simulink model "ofdmexample1"  (R2017a)
settings: Solver=FixedStepDiscrete  StartTime=0.0  StopTime=0.1  RelTol=1e-3
PostLoadFcn:
  | prm80216d.blkh = []; prm80216d.action = 'init';
  | commwman80216d_init(prm80216d.blkh, prm80216d.action);
  | if isempty(ans), clear ans; end
StartFcn:
  | if isempty(ans), clear ans; end
undefined symbols (not defined in the file): idx, magnitude
libraries: commwman80216d_lib x49, dspsigops x24, commcnvcod2 x14, dspindex x4, commdigbbndpm3 x3, dspsolvers x2, simulink x2, commrflib2 x2, commofdm x2, commsink2 x1, commblksprivate x1, dspmtrx3 x1
(part 1 of 2)
Description:
  | IEEE 802.16-2004 WirelessMAN-OFDM PHY Downlink model
settings Model: FPTRunName=Active  ExtModeAutoUpdateStatusClock=off  Creator=The MathWorks, Inc.  LastModifiedBy=max
settings DataIOCC: LimitDataPoints=on  SaveFormat=Array
settings OptimizationCC: ExpressionDepthLimit=2147483647  InitFltsAndDblsToZero=on  EfficientMapNaN2IntZero=off  LifeSpan=inf
settings DebuggingCC: UnderspecifiedInitializationDetection=Classic  MergeDetectMultiDrivingBlocksExec=none  FcnCallInpInsideContextMsg=warning  AllowSymbolicDim=off  StateNameClashWarn=warning  SFUnexpectedBacktrackingDiag=warning  SFNoUnconditionalDefaultTransitionDiag=warning  SFExecutionAtInitializationDiag=none
settings HardwareCC: ProdBitPerPointer=32  ProdBitPerSizeT=32  ProdBitPerPtrDiffT=32  ProdLargestAtomicFloat=None  ProdIntDivRoundTo=Undefined  ProdEndianess=Unspecified  ProdWordSize=32  ProdHWDeviceType=32-bit Generic
settings ModelReferenceCC: PropagateSignalLabelsOutOfModel=off
settings RTWCC: RetainRTWFile=on
settings GRTTargetCC: TargetFcnLib=ansi_tfl_tmw_new.mat  TargetLangStandard=C89/C90 (ANSI)  GeneratePreprocessorConditionals=Disable all  CombineOutputUpdateFcns=off  GRTInterface=on
settings ConfigComp: CovMetricSettings=dw  CovHtmlReporting=on  CovSaveCumulativeToWorkspaceVar=on  CovSaveSingleToWorkspaceVar=on  CovExternalEMLEnable=off  CovSFcnEnable=off

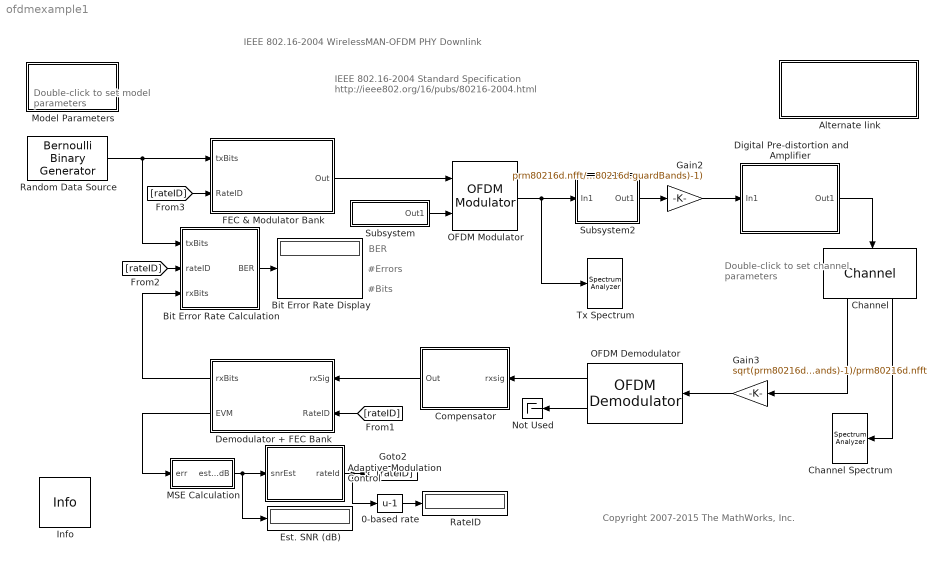
== system ofdmexample1 ==
  note: IEEE 802.16-2004 WirelessMAN-OFDM PHY Downlink
  note: BER
  note: #Bits
  note: #Errors
  note: Double-click to set
      | channel parameters
  note: Double-click to
      | set model parameters
  note: IEEE 802.16-2004 Standard Specification
      | http://ieee802.org/16/pubs/80216-2004.html
  note: Copyright 2007-2015 The MathWorks, Inc.
  0-based rate : Bias  Bias=-1
  Adaptive Modulation Control : Subsystem  mask{thres=prm80216d.thresholds}
      mask prompts: thres "Low-SNR thresholds (dB):"
      mask init:
      | snrUp = [thres inf];
      | snrDown = [-inf thres];
      mask Display: disp('Adaptive\nRate\nControl')
  Alternate link : Subsystem
      settings: OpenFcn=commwman80216dstbc;
      mask Display: disp('Double-click to open\n link model with\nSpace-Time Block Coding');
  Bit Error Rate Calculation : Subsystem
      mask Display: disp('Bit Error Rate\nCalculation');
  Bit Error Rate Display : Display
  Channel : commwman80216d_lib/Channel  fadingMode=Frequency-selective fading  K=4  maxDoppler=0.5  pathDelays=[0 0.4 0.9]*1e-6  pathGains=[0 -15 -20]  SNRdB=30
      settings: SourceProductName=Communications System Toolbox  SourceProductBaseCode=CM
  Channel Spectrum : SpectrumAnalyzer
  Compensator : Subsystem
      mask Display: disp('Gain & Phase\nCompensator');
  Demodulator + FEC Bank : Subsystem
      mask Display: disp('Demodulator\n& FEC Bank');
  Digital Pre-distortion and Amplifier : Subsystem
      mask Display: disp('Digital\nPre-Distortion and\nNonlinear\nAmplifier')
  Est. SNR (dB) : Display
  FEC & Modulator Bank : Subsystem
      mask Display: disp('FEC & \nModulator Bank');
  Gain2 : Gain  Gain=prm80216d.nfft/sqrt(prm80216d.nfft-sum(prm80216d.guardBands)-1)
  Gain3 : Gain  Gain=sqrt(prm80216d.nfft-sum(prm80216d.guardBands)-1)/prm80216d.nfft
  Info : commblksprivate/Info  SystemSampleTime=-1
      settings: SourceProductName=Communications System Toolbox  SourceProductBaseCode=CM
  MSE Calculation : Subsystem
      mask Display: disp('SNR\nEstimation')
  Model Parameters : Subsystem  mask(Model Parameters){chanBW=3.5, numSym=1, g=1/8, nonlinCtrl=Disabled, dpdCtrl=Disabled, thresh=[4 10 12 19 22 28]}
      mask prompts: chanBW "Channel bandwidth (MHz):"; numSym "Number of OFDM symbols per burst:"; g "Cyclic prefix factor (G):"; nonlinCtrl "Amplifier nonlinearity:"; dpdCtrl "Digital pre-distortion:"; thresh "Low SNR thresholds for rate control (dB):"
      mask help: Specifies model parameters for a simulation run.
      mask init:
      | numPreSym = 1; % number of preamble OFDM symbols
      | 
      | % If the nonlinearity is turned off, then turn off the digital
      | % pre-distortion
      | if nonlinCtrl == 1  % disabled
      |     dpdCtrl = 1;
      | end
      | 
      | myException = commwman80216d_init(gcbh, 'init', chanBW, ...
      |     numSym, numPreSym, g, thresh);
      | 
      | if ~isempty(myException)
      |     errordlg(myException.msg);
      | end
      mask Help: helpview(commdhelp);
      mask TypeOptions g: 1/4 | 1/8 | 1/16 | 1/32
      mask TypeOptions nonlinCtrl: Disabled | Moderate (correctable by pre-distortion) | Severe (uncorrectable by pre-distortion)
      mask Callback nonlinCtrl: commwman80216d_init(gcbh, 'cbShowHidePreDistortion');
      mask TypeOptions dpdCtrl: Disabled | Enabled
      mask Display: disp('Model\nParameters');
  Not Used : Terminator
  OFDM Demodulator : commofdm/OFDM Demodulator  FFTLength=prm80216d.nfft  NumGuardBandCarriers=prm80216d.guardBands  RemoveDCCarrier=on  PilotOutputPort=on  PilotCarrierIndices=prm80216d.pilotIndices + prm80216d.nfft/2 + 1  CyclicPrefixLength=prm80216d.CPLen  NumSymbols=prm80216d.totOFDMSym  NumReceiveAntennas=1  SimulateUsing=Interpreted execution
      settings: SourceProductName=Communications System Toolbox  SourceProductBaseCode=CM
  OFDM Modulator : commofdm/OFDM Modulator  FFTLength=prm80216d.nfft  NumGuardBandCarriers=prm80216d.guardBands  InsertDCNull=on  PilotInputPort=on  PilotCarrierIndices=prm80216d.pilotIndices + prm80216d.nfft/2 + 1  CyclicPrefixLength=prm80216d.CPLen  Windowing=off  WindowLength=1  NumSymbols=prm80216d.numOFDMSymbols  NumTransmitAntennas=1  SimulateUsing=Interpreted execution
      settings: SourceProductName=Communications System Toolbox  SourceProductBaseCode=CM
  Random Data Source : commrandsrc3/Bernoulli Binary Generator  ProbabilityOfZero=0.5  SeedSource=Parameter  Seed=61  SampleTime=prm80216d.minBitPeriod  SamplesPerFrame=prm80216d.maxUncBitsPerBlk*prm80216d.numOFDMSymbols  OutputDataType=boolean  SimulateUsing=Interpreted execution
  RateID : Display
  Subsystem : Subsystem
      mask Display: disp('Pilot')
  Subsystem2 : Subsystem
      mask Display: disp('Preamble\nPacking');
  Tx Spectrum : SpectrumAnalyzer
  wires:
  Gain2/1 -> Digital Pre-distortion and Amplifier/1(In1)
  Random Data Source/1 -> Bit Error Rate Calculation/1(txBits), FEC & Modulator Bank/1(txBits)
  Bit Error Rate Calculation/1(BER) -> Bit Error Rate Display/1
  Demodulator + FEC Bank/2(EVM) -> MSE Calculation/1(err)
  [rateID] -> FEC & Modulator Bank/2(RateID)
  [rateID] -> Demodulator + FEC Bank/2(RateID)
  [rateID] -> Bit Error Rate Calculation/2(rateID)
  Demodulator + FEC Bank/1(rxBits) -> Bit Error Rate Calculation/3(rxBits)
  Adaptive Modulation Control/1(rateId) -> [rateID], 0-based rate/1
  MSE Calculation/1(estSNRdB) -> Adaptive Modulation Control/1(snrEst), Est. SNR (dB)/1
  0-based rate/1 -> RateID/1
  Digital Pre-distortion and Amplifier/1(Out1) -> Channel/1
  Channel/1 -> Gain3/1
  Channel/2 -> Channel Spectrum/1
  Gain3/1 -> OFDM Demodulator/1
  OFDM Demodulator/1 -> Compensator/1(rxsig)
  OFDM Demodulator/2 -> Not Used/1
  Subsystem/1(Out1) -> OFDM Modulator/2
  OFDM Modulator/1 -> Subsystem2/1(In1), Tx Spectrum/1
  FEC & Modulator Bank/1(Out) -> OFDM Modulator/1
  Compensator/1(Out) -> Demodulator + FEC Bank/1(rxSig)
  Subsystem2/1(Out1) -> Gain2/1

== system ofdmexample1/Adaptive Modulation Control ==
  note: dec by 1
  note: inc by 1
  snrEst : Inport
  Add1 : Sum  Inputs=+-+  OutDataTypeStr=double
  Integer Delay : Delay  DelayLength=1  InitialCondition=1 % rateID 0 => BPSK
  Relational Operator : RelationalOperator  Operator=>  RndMeth=Nearest
  Relational Operator1 : RelationalOperator  Operator=<=  RndMeth=Nearest
  SNR down threshold : commwman80216d_lib/Select Value  vector=snrDown
      settings: SourceProductName=Communications System Toolbox  SourceProductBaseCode=CM
  SNR up threshold : commwman80216d_lib/Select Value  vector=snrUp
      settings: SourceProductName=Communications System Toolbox  SourceProductBaseCode=CM
  rateId : Outport
  wires:
  Add1/1 -> Integer Delay/1
  SNR down threshold/1 -> Relational Operator1/2
  SNR up threshold/1 -> Relational Operator/2
  Integer Delay/1 -> rateId/1, SNR up threshold/1, SNR down threshold/1, Add1/3
  Relational Operator1/1 -> Add1/2
  Relational Operator/1 -> Add1/1
  snrEst/1 -> Relational Operator1/1, Relational Operator/1

== system ofdmexample1/Alternate link ==

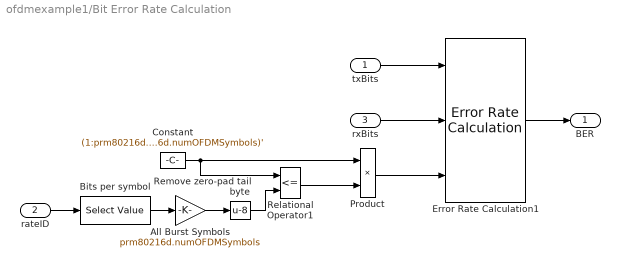
== system ofdmexample1/Bit Error Rate Calculation ==
  txBits : Inport
  rateID : Inport  Port=2
  rxBits : Inport  Port=3
  All Burst Symbols : Gain  Gain=prm80216d.numOFDMSymbols
  Bits per symbol : commwman80216d_lib/Select Value  vector=prm80216d.uncBlkSize*8
      settings: SourceProductName=Communications System Toolbox  SourceProductBaseCode=CM
  Constant : Constant  Value=(1:prm80216d.maxUncBitsPerBlk*prm80216d.numOFDMSymbols)'  VectorParams1D=off
  Error Rate Calculation1 : commsink2/Error Rate Calculation  N=0  st_delay=0  cp_mode=Select samples from port  subframe=1:(idx*8*prm80216d.numOFDMSymbols - 8)  PMode=Port  WsName=ErrorVec  RsMode2=off  stop=off  numErr=inf  maxBits=5e5
  Product : Product  SaturateOnIntegerOverflow=on  OutDataTypeStr=Inherit: Same as first input
  Relational Operator1 : RelationalOperator  Operator=<=  OutDataTypeStr=float('double')  RndMeth=Nearest  InputSameDT=on
  Remove zero-pad tail byte : Bias  Bias=-8
  BER : Outport
  wires:
  txBits/1 -> Error Rate Calculation1/1
  Error Rate Calculation1/1 -> BER/1
  rxBits/1 -> Error Rate Calculation1/2
  rateID/1 -> Bits per symbol/1
  Relational Operator1/1 -> Product/2
  Constant/1 -> Product/1, Relational Operator1/1
  All Burst Symbols/1 -> Remove zero-pad tail byte/1
  Product/1 -> Error Rate Calculation1/3
  Bits per symbol/1 -> All Burst Symbols/1
  Remove zero-pad tail byte/1 -> Relational Operator1/2

== system ofdmexample1/Compensator ==
  rxsig : Inport
  Compensator : Subsystem
      mask init:
      | a = [1:100; 1:100];
      mask Display: disp('Gain & Phase\nCompensator')
  Extract Nonzero Preamble Subcarriers : dspindex/Multiport Selector  rowsOrCols=Rows  idxCellArray=prm80216d.nonzeroPreambleIdxTx1  idxErrMode=Clip Index
  Training Preamble : Constant  Value=prm80216d.preambleTx1  VectorParams1D=off
  Out : Outport
  wires:
  Training Preamble/1 -> Extract Nonzero Preamble Subcarriers/1
  rxsig/1 -> Compensator/1(rxsig)
  Compensator/1(out) -> Out/1
  Extract Nonzero Preamble Subcarriers/1 -> Compensator/2(trainsig)

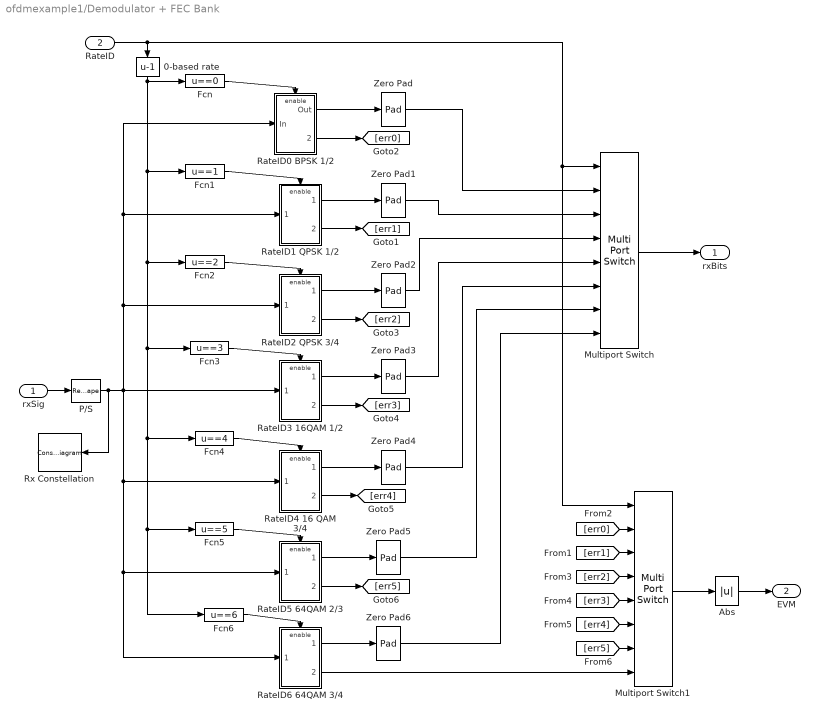
== system ofdmexample1/Demodulator + FEC Bank ==
  rxSig : Inport
  RateID : Inport  Port=2
  0-based rate : Bias  Bias=-1
  Abs : Abs  SaturateOnIntegerOverflow=on
  Fcn : Fcn  Expr=u==0
  Fcn1 : Fcn  Expr=u==1
  Fcn2 : Fcn  Expr=u==2
  Fcn3 : Fcn  Expr=u==3
  Fcn4 : Fcn  Expr=u==4
  Fcn5 : Fcn  Expr=u==5
  Fcn6 : Fcn  Expr=u==6
  Multiport Switch : MultiPortSwitch  Inputs=7  SaturateOnIntegerOverflow=on
  Multiport Switch1 : MultiPortSwitch  Inputs=7  SaturateOnIntegerOverflow=on
  P/S : Reshape  OutputDimensionality=Column vector (2-D)  OutputDimensions=[prm80216d.numDataSym, prm80216d.numOFDMSymbols]
  RateID0 BPSK 1/2 : Subsystem
  RateID1 QPSK 1/2 : Subsystem
  RateID2 QPSK 3/4 : Subsystem
  RateID3 16QAM 1/2 : Subsystem
  RateID4 16 QAM 3/4 : Subsystem
  RateID5 64QAM 2/3 : Subsystem
  RateID6 64QAM 3/4 : Subsystem
  Rx Constellation : ConstellationDiagram  Tag=ScatterPlot
  Zero Pad{,1..6} (7 alike) : dspsigops/Pad  padAlong=Columns  dimsToPad=1  valSrc=Specify via dialog  padVal=0  spec=Output size  padNumOutRowsSpecMethod=User-specified  numOutRows=prm80216d.maxUncBitsPerBlk*prm80216d.numOFDMSymbols  padNumOutColsSpecMethod=User-specified  numOutCols=1  isVarDimsMode=off  padBeginning=0  padEnd=0  outSizeMode=User-specified  outSize=1  padSigAt=End  trunc_flag=None  roundingMode=Floor  overflowMode=off  truncOrWrapMode=Truncate  wrap_flag=None
      settings: AttributesFormatString=\n  SourceProductName=DSP System Toolbox  SourceProductBaseCode=DS
  rxBits : Outport
  EVM : Outport  Port=2
  wires:
  RateID/1 -> Multiport Switch/1, Multiport Switch1/1, 0-based rate/1
  Multiport Switch/1 -> rxBits/1
  RateID0 BPSK 1/2/1(Out) -> Zero Pad/1
  RateID1 QPSK 1/2/1(Out1) -> Zero Pad1/1
  RateID2 QPSK 3/4/1(Out2) -> Zero Pad2/1
  RateID3 16QAM 1/2/1(Out3) -> Zero Pad3/1
  RateID4 16 QAM 3/4/1(Out4) -> Zero Pad4/1
  RateID5 64QAM 2/3/1(Out5) -> Zero Pad5/1
  RateID6 64QAM 3/4/1(Out6) -> Zero Pad6/1
  Fcn/1 -> RateID0 BPSK 1/2/Enable
  Fcn1/1 -> RateID1 QPSK 1/2/Enable
  Fcn2/1 -> RateID2 QPSK 3/4/Enable
  Fcn3/1 -> RateID3 16QAM 1/2/Enable
  Fcn4/1 -> RateID4 16 QAM 3/4/Enable
  Fcn5/1 -> RateID5 64QAM 2/3/Enable
  Fcn6/1 -> RateID6 64QAM 3/4/Enable
  Zero Pad/1 -> Multiport Switch/2
  Zero Pad2/1 -> Multiport Switch/4
  Zero Pad3/1 -> Multiport Switch/5
  Zero Pad4/1 -> Multiport Switch/6
  Zero Pad5/1 -> Multiport Switch/7
  Zero Pad6/1 -> Multiport Switch/8
  Multiport Switch1/1 -> Abs/1
  RateID6 64QAM 3/4/2(symerr) -> Multiport Switch1/8
  Abs/1 -> EVM/1
  0-based rate/1 -> Fcn/1, Fcn1/1, Fcn2/1, Fcn3/1, Fcn4/1, Fcn5/1, Fcn6/1
  RateID0 BPSK 1/2/2(symerr) -> [err0]
  RateID1 QPSK 1/2/2(symerr) -> [err1]
  RateID2 QPSK 3/4/2(symerr) -> [err2]
  RateID3 16QAM 1/2/2(symerr) -> [err3]
  RateID4 16 QAM 3/4/2(symerr) -> [err4]
  RateID5 64QAM 2/3/2(symerr) -> [err5]
  [err0] -> Multiport Switch1/2
  [err1] -> Multiport Switch1/3
  [err2] -> Multiport Switch1/4
  [err3] -> Multiport Switch1/5
  [err4] -> Multiport Switch1/6
  [err5] -> Multiport Switch1/7
  Zero Pad1/1 -> Multiport Switch/3
  rxSig/1 -> P/S/1
  P/S/1 -> Rx Constellation/1, RateID4 16 QAM 3/4/1(In4), RateID5 64QAM 2/3/1(In5), RateID6 64QAM 3/4/1(In6), RateID0 BPSK 1/2/1(In), RateID1 QPSK 1/2/1(In1), RateID2 QPSK 3/4/1(In2), RateID3 16QAM 1/2/1(In3)

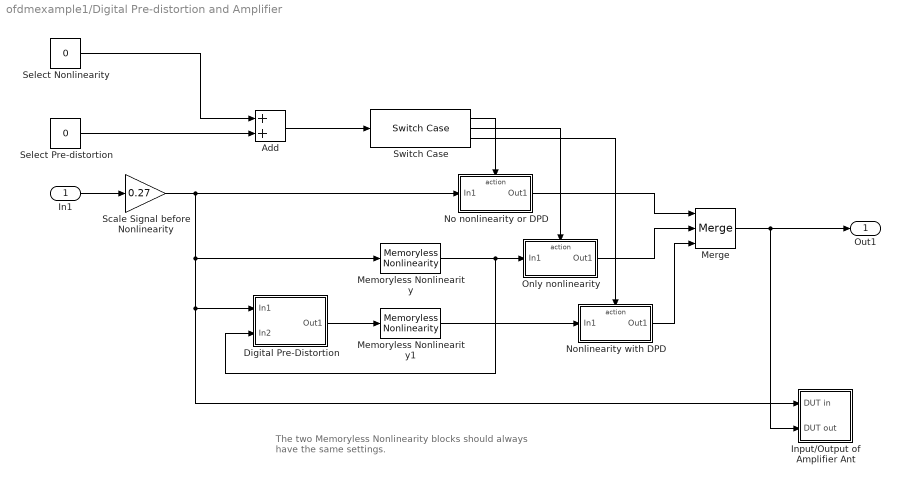
== system ofdmexample1/Digital Pre-distortion and Amplifier ==
  note: The two Memoryless Nonlinearity blocks should always
      | have the same settings.
  In1 : Inport
  Add : Sum
  Digital Pre-Distortion : Subsystem
      mask Display: disp('Digital\nPre-Distortion')
  Input/Output of Amplifier Ant : Subsystem
  Memoryless Nonlinearity : commrflib2/Memoryless Nonlinearity  model_select=Saleh model  linGaindB=0  GindB=0  iip3=30  am2pm=10  LPwrLimAMPM=10  UPwrLimAMPM=inf  amam=[2.1587 1.1517]  ampm=[4.0033 9.1040]  x=[8.1081 1.5413 6.5202 -0.0718]  y=[4.6645 2.0965 10.88 -0.003]  p=0.5  GoutdB=0  vsat=1
      settings: SourceProductName=Communications System Toolbox  SourceProductBaseCode=CM
  Memoryless Nonlinearity1 : commrflib2/Memoryless Nonlinearity  model_select=Saleh model  linGaindB=0  GindB=0  iip3=30  am2pm=10  LPwrLimAMPM=10  UPwrLimAMPM=inf  amam=[2.1587 1.1517]  ampm=[4.0033 9.1040]  x=[8.1081 1.5413 6.5202 -0.0718]  y=[4.6645 2.0965 10.88 -0.003]  p=0.5  GoutdB=0  vsat=1
      settings: SourceProductName=Communications System Toolbox  SourceProductBaseCode=CM
  Merge : Merge  Inputs=3
  No nonlinearity or DPD : Subsystem  TreatAsAtomicUnit=on
  Nonlinearity with DPD : Subsystem  TreatAsAtomicUnit=on
  Only nonlinearity : Subsystem  TreatAsAtomicUnit=on
  Scale Signal before Nonlinearity : Gain  Gain=0.27
  Select Nonlinearity : Constant  Value=0
  Select Pre-distortion : Constant  Value=0
  Switch Case : SwitchCase  CaseConditions={0,1,2}  ShowDefaultCase=off
  Out1 : Outport
  wires:
  Scale Signal before Nonlinearity/1 -> No nonlinearity or DPD/1(In1), Input/Output of Amplifier Ant/1(DUT in), Digital Pre-Distortion/1(In1), Memoryless Nonlinearity/1
  Digital Pre-Distortion/1(Out1) -> Memoryless Nonlinearity1/1
  Select Pre-distortion/1 -> Add/2
  Add/1 -> Switch Case/1
  Select Nonlinearity/1 -> Add/1
  In1/1 -> Scale Signal before Nonlinearity/1
  Memoryless Nonlinearity1/1 -> Nonlinearity with DPD/1(In1)
  Memoryless Nonlinearity/1 -> Only nonlinearity/1(In1), Digital Pre-Distortion/2(In2)
  Merge/1 -> Input/Output of Amplifier Ant/2(DUT out), Out1/1
  Switch Case/1 -> No nonlinearity or DPD/Action
  Switch Case/2 -> Only nonlinearity/Action
  Switch Case/3 -> Nonlinearity with DPD/Action
  No nonlinearity or DPD/1(Out1) -> Merge/1
  Only nonlinearity/1(Out1) -> Merge/2
  Nonlinearity with DPD/1(Out1) -> Merge/3

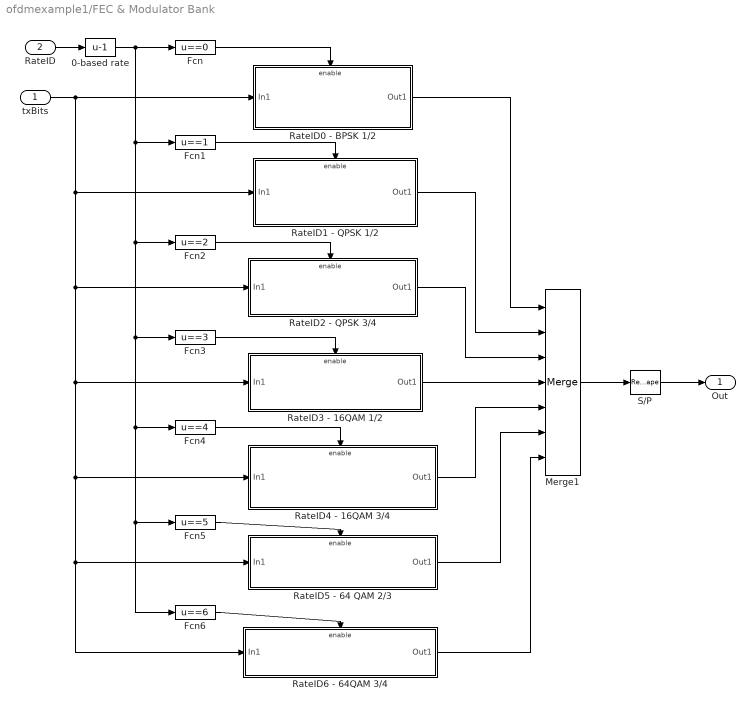
== system ofdmexample1/FEC & Modulator Bank ==
  txBits : Inport
  RateID : Inport  Port=2
  0-based rate : Bias  Bias=-1
  Fcn : Fcn  Expr=u==0
  Fcn1 : Fcn  Expr=u==1
  Fcn2 : Fcn  Expr=u==2
  Fcn3 : Fcn  Expr=u==3
  Fcn4 : Fcn  Expr=u==4
  Fcn5 : Fcn  Expr=u==5
  Fcn6 : Fcn  Expr=u==6
  Merge1 : Merge  Inputs=7
  RateID0 - BPSK 1/2 : Subsystem
  RateID1 - QPSK 1/2 : Subsystem
  RateID2 - QPSK 3/4 : Subsystem
  RateID3 - 16QAM 1/2 : Subsystem
  RateID4 - 16QAM 3/4 : Subsystem
  RateID5 - 64 QAM 2/3 : Subsystem
  RateID6 - 64QAM 3/4 : Subsystem
  S/P : Reshape  OutputDimensionality=Customize  OutputDimensions=[prm80216d.numDataCarriers, prm80216d.numOFDMSymbols]
  Out : Outport
  wires:
  RateID0 - BPSK 1/2/1(Out1) -> Merge1/1
  RateID1 - QPSK 1/2/1(Out1) -> Merge1/2
  RateID2 - QPSK 3/4/1(Out1) -> Merge1/3
  RateID3 - 16QAM 1/2/1(Out1) -> Merge1/4
  RateID4 - 16QAM 3/4/1(Out1) -> Merge1/5
  RateID5 - 64 QAM 2/3/1(Out1) -> Merge1/6
  RateID6 - 64QAM 3/4/1(Out1) -> Merge1/7
  txBits/1 -> RateID5 - 64 QAM 2/3/1(In1), RateID6 - 64QAM 3/4/1(In1), RateID4 - 16QAM 3/4/1(In1), RateID3 - 16QAM 1/2/1(In1), RateID2 - QPSK 3/4/1(In1), RateID1 - QPSK 1/2/1(In1), RateID0 - BPSK 1/2/1(In1)
  RateID/1 -> 0-based rate/1
  Fcn/1 -> RateID0 - BPSK 1/2/Enable
  Fcn1/1 -> RateID1 - QPSK 1/2/Enable
  Fcn2/1 -> RateID2 - QPSK 3/4/Enable
  Fcn3/1 -> RateID3 - 16QAM 1/2/Enable
  Fcn4/1 -> RateID4 - 16QAM 3/4/Enable
  Fcn5/1 -> RateID5 - 64 QAM 2/3/Enable
  Fcn6/1 -> RateID6 - 64QAM 3/4/Enable
  0-based rate/1 -> Fcn4/1, Fcn5/1, Fcn6/1, Fcn3/1, Fcn2/1, Fcn1/1, Fcn/1
  Merge1/1 -> S/P/1
  S/P/1 -> Out/1

== system ofdmexample1/MSE Calculation ==
  err : Inport
  Math Function2 : Math  Operator=reciprocal  SaturateOnIntegerOverflow=on
  Matrix Square : dspmtrx3/Matrix Square  OutMin=[]  OutMax=[]
      settings: SourceProductName=DSP System Toolbox  SourceProductBaseCode=DS
  RMS : dspstat3/RMS  run=off  directionMode=Each column  dimension=1  InputProcessing=Columns as channels (frame based)  reset_popup=None
  dB Conversion : dspmathops/dB Conversion  dBtype=dB  intype=Power  R=1  fuzz=on
      settings: SourceProductName=DSP System Toolbox
  estSNRdB : Outport
  wires:
  dB Conversion/1 -> estSNRdB/1
  err/1 -> RMS/1
  RMS/1 -> Matrix Square/1
  Math Function2/1 -> dB Conversion/1
  Matrix Square/1 -> Math Function2/1

== system ofdmexample1/Model Parameters ==
  note: This subsystem is empty.
      | It is used for setting parameter values (in the mask).

== system ofdmexample1/Subsystem ==
  Gain{,1,3..4} (4 alike) : Gain  Gain=-1
  Input Packing : Concatenate  NumInputs=8  Mode=Multidimensional array
  Pilots : commwman80216d_lib/Pilot Generator  link=Downlink  ts=prm80216d.maxUncBitsPerBlk*prm80216d.minBitPeriod  numSym=prm80216d.numOFDMSymbols  shift=prm80216d.numPreamOFDMSymbols
      settings: SourceProductName=Communications System Toolbox  SourceProductBaseCode=CM
  Out1 : Outport
  wires:
  Gain/1 -> Input Packing/4
  Pilots/1 -> Input Packing/1, Gain1/1, Input Packing/3, Gain/1, Gain3/1, Gain4/1, Input Packing/7, Input Packing/8
  Gain3/1 -> Input Packing/5
  Gain1/1 -> Input Packing/2
  Gain4/1 -> Input Packing/6
  Input Packing/1 -> Out1/1

== system ofdmexample1/Subsystem2 ==
  In1 : Inport
  Insert Preamble : Concatenate  Mode=Multidimensional array
  Subsystem1 : Subsystem
      mask Display: disp('Preamble')
  Out1 : Outport
  wires:
  In1/1 -> Insert Preamble/2
  Insert Preamble/1 -> Out1/1
  Subsystem1/1(Out) -> Insert Preamble/1

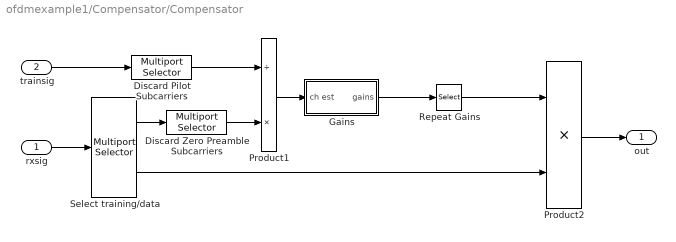
== system ofdmexample1/Compensator/Compensator ==
  rxsig : Inport
  trainsig : Inport  Port=2
  Discard Pilot Subcarriers : dspindex/Multiport Selector  rowsOrCols=Rows  idxCellArray=prm80216d.preambleEqIdxTx1  idxErrMode=Clip Index
  Discard Zero Preamble Subcarriers : dspindex/Multiport Selector  rowsOrCols=Rows  idxCellArray=prm80216d.dataEqIdxTx1  idxErrMode=Clip Index
  Gains : Subsystem
  Product1 : Product  Inputs=/*  SaturateOnIntegerOverflow=on  OutDataTypeStr=Inherit: Same as first input
  Product2 : Product  Inputs=**  SaturateOnIntegerOverflow=on  OutDataTypeStr=Inherit: Same as first input
  Repeat Gains : Selector  NumberOfDimensions=2  InputPortWidth=53  IndexOptions=Index vector (dialog),Select all  Indices=kron(1:prm80216d.numDataCarriers/2, [1 1]),-1  OutputSizes=1
  Select training/data : dspindex/Multiport Selector  rowsOrCols=Columns  idxCellArray={1:prm80216d.numPreamOFDMSymbols, prm80216d.numPreamOFDMSymbols+1:prm80216d.totOFDMSym}  idxErrMode=Clip Index
  out : Outport
  wires:
  Select training/data/1 -> Discard Zero Preamble Subcarriers/1
  Product2/1 -> out/1
  Product1/1 -> Gains/1(ch est)
  Gains/1(gains) -> Repeat Gains/1
  rxsig/1 -> Select training/data/1
  Repeat Gains/1 -> Product2/1
  Select training/data/2 -> Product2/2
  trainsig/1 -> Discard Pilot Subcarriers/1
  Discard Zero Preamble Subcarriers/1 -> Product1/2
  Discard Pilot Subcarriers/1 -> Product1/1

== system ofdmexample1/Demodulator + FEC Bank/RateID0 BPSK 1//2 ==
  In : Inport
  Enable : EnablePort  StatesWhenEnabling=reset  PropagateVarSize=During execution
  BPSK Demodulator : commdigbbndpm3/BPSK Demodulator Baseband  DecType=Hard decision  VarSource=Dialog  Variance=1  Ph=0  outDtype=boolean  derotateFactorWordLen=16  derotateFactorDataTypeStr=Inherit: Same word length as input  derotateFactorLastDataTypeStr=Inherit: Same word length as input
  BPSK Modulator : commdigbbndpm3/BPSK Modulator Baseband  Ph=0  outDtype=double  outWordLen=16  outUDDataType=sfix(16)  outFracLenMode=Best precision  outFracLen=15  outDataTypeStr=double  outLastDataTypeStr=double
  Deinterleaver : commwman80216d_lib/Deinterleaver  numSubCh=16  Ncbps1=192  Ncbps2=96  Ncbps3=48  Ncbps4=24  Ncbps5=12  Ncpc=1  numSym=prm80216d.numOFDMSymbols
      settings: SourceProductName=Communications System Toolbox  SourceProductBaseCode=CM
  Sum : Sum  Inputs=|+-  SaturateOnIntegerOverflow=on
  Viterbi Decoder : commcnvcod2/Viterbi Decoder  trellis=poly2trellis(7, [171 133])  isPunctured=off  punctureVector=reshape([1 0 1 0 1;1 1 0 1 0],10,1)  erasures=off  dectype=Hard decision  nsdecb=4  runSigValErrCheck=off  tbdepth=34  opmode=Truncated  reset=off  delayedResetAction=off  smWordLength=16  outDataType=boolean
      settings: SourceProductName=Communications System Toolbox  SourceProductBaseCode=CM
  Out : Outport
  symerr : Outport  Port=2  OutputWhenDisabled=reset  InitialOutput=0
  wires:
  Sum/1 -> symerr/1
  In/1 -> BPSK Demodulator/1, Sum/2
  BPSK Demodulator/1 -> Deinterleaver/1, BPSK Modulator/1
  Deinterleaver/1 -> Viterbi Decoder/1
  Viterbi Decoder/1 -> Out/1
  BPSK Modulator/1 -> Sum/1

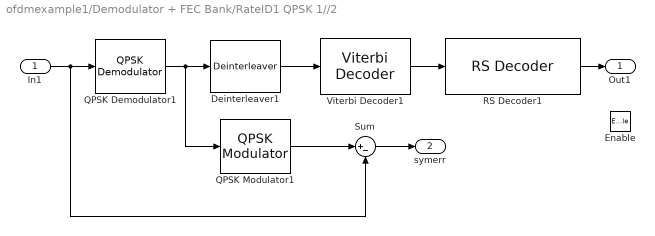
== system ofdmexample1/Demodulator + FEC Bank/RateID1 QPSK 1//2 ==
  In1 : Inport
  Enable : EnablePort  StatesWhenEnabling=reset  PropagateVarSize=During execution
  Deinterleaver1 : commwman80216d_lib/Deinterleaver  numSubCh=16  Ncbps1=384  Ncbps2=96  Ncbps3=48  Ncbps4=24  Ncbps5=12  Ncpc=2  numSym=prm80216d.numOFDMSymbols
      settings: SourceProductName=Communications System Toolbox  SourceProductBaseCode=CM
  QPSK Demodulator1 : commwman80216d_lib/QPSK Demodulator  SystemSampleTime=-1
      settings: SourceProductName=Communications System Toolbox  SourceProductBaseCode=CM
  QPSK Modulator1 : commwman80216d_lib/QPSK Modulator  SystemSampleTime=-1
      settings: SourceProductName=Communications System Toolbox  SourceProductBaseCode=CM
  RS Decoder1 : commwman80216d_lib/RS Decoder  N=32  K=24  numSym=prm80216d.numOFDMSymbols
      settings: SourceProductName=Communications System Toolbox  SourceProductBaseCode=CM
  Sum : Sum  Inputs=|+-  SaturateOnIntegerOverflow=on
  Viterbi Decoder1 : commcnvcod2/Viterbi Decoder  trellis=poly2trellis(7, [171 133])  isPunctured=on  punctureVector=reshape([1 0;1 1],4,1)  erasures=off  dectype=Hard decision  nsdecb=4  runSigValErrCheck=off  tbdepth=34  opmode=Truncated  reset=off  delayedResetAction=off  smWordLength=16  outDataType=boolean
      settings: SourceProductName=Communications System Toolbox  SourceProductBaseCode=CM
  Out1 : Outport
  symerr : Outport  Port=2  OutputWhenDisabled=reset  InitialOutput=0
  wires:
  In1/1 -> QPSK Demodulator1/1, Sum/2
  QPSK Demodulator1/1 -> Deinterleaver1/1, QPSK Modulator1/1
  Deinterleaver1/1 -> Viterbi Decoder1/1
  Viterbi Decoder1/1 -> RS Decoder1/1
  RS Decoder1/1 -> Out1/1
  Sum/1 -> symerr/1
  QPSK Modulator1/1 -> Sum/1

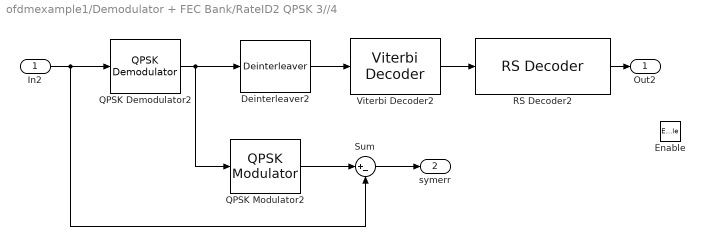
== system ofdmexample1/Demodulator + FEC Bank/RateID2 QPSK 3//4 ==
  In2 : Inport
  Enable : EnablePort  StatesWhenEnabling=reset  PropagateVarSize=During execution
  Deinterleaver2 : commwman80216d_lib/Deinterleaver  numSubCh=16  Ncbps1=384  Ncbps2=96  Ncbps3=48  Ncbps4=24  Ncbps5=12  Ncpc=2  numSym=prm80216d.numOFDMSymbols
      settings: SourceProductName=Communications System Toolbox  SourceProductBaseCode=CM
  QPSK Demodulator2 : commwman80216d_lib/QPSK Demodulator  SystemSampleTime=-1
      settings: SourceProductName=Communications System Toolbox  SourceProductBaseCode=CM
  QPSK Modulator2 : commwman80216d_lib/QPSK Modulator  SystemSampleTime=-1
      settings: SourceProductName=Communications System Toolbox  SourceProductBaseCode=CM
  RS Decoder2 : commwman80216d_lib/RS Decoder  N=40  K=36  numSym=prm80216d.numOFDMSymbols
      settings: SourceProductName=Communications System Toolbox  SourceProductBaseCode=CM
  Sum : Sum  Inputs=|+-  SaturateOnIntegerOverflow=on
  Viterbi Decoder2 : commcnvcod2/Viterbi Decoder  trellis=poly2trellis(7, [171 133])  isPunctured=on  punctureVector=reshape([1 0 1 0 1;1 1 0 1 0],10,1)  erasures=off  dectype=Hard decision  nsdecb=4  runSigValErrCheck=off  tbdepth=34  opmode=Truncated  reset=off  delayedResetAction=off  smWordLength=16  outDataType=boolean
      settings: SourceProductName=Communications System Toolbox  SourceProductBaseCode=CM
  Out2 : Outport
  symerr : Outport  Port=2  OutputWhenDisabled=reset  InitialOutput=0
  wires:
  In2/1 -> QPSK Demodulator2/1, Sum/2
  QPSK Demodulator2/1 -> Deinterleaver2/1, QPSK Modulator2/1
  Deinterleaver2/1 -> Viterbi Decoder2/1
  Viterbi Decoder2/1 -> RS Decoder2/1
  RS Decoder2/1 -> Out2/1
  QPSK Modulator2/1 -> Sum/1
  Sum/1 -> symerr/1

== system ofdmexample1/Demodulator + FEC Bank/RateID3 16QAM 1//2 ==
  In3 : Inport
  Enable : EnablePort  StatesWhenEnabling=reset  PropagateVarSize=During execution
  16-QAM Demodulator3 : commwman80216d_lib/16-QAM Demodulator  SystemSampleTime=-1
      settings: SourceProductName=Communications System Toolbox  SourceProductBaseCode=CM
  16-QAM Modulator3 : commwman80216d_lib/16-QAM Modulator  SystemSampleTime=-1
      settings: SourceProductName=Communications System Toolbox  SourceProductBaseCode=CM
  Deinterleaver3 : commwman80216d_lib/Deinterleaver  numSubCh=16  Ncbps1=768  Ncbps2=96  Ncbps3=48  Ncbps4=24  Ncbps5=12  Ncpc=4  numSym=prm80216d.numOFDMSymbols
      settings: SourceProductName=Communications System Toolbox  SourceProductBaseCode=CM
  RS Decoder3 : commwman80216d_lib/RS Decoder  N=64  K=48  numSym=prm80216d.numOFDMSymbols
      settings: SourceProductName=Communications System Toolbox  SourceProductBaseCode=CM
  Sum : Sum  Inputs=|+-  SaturateOnIntegerOverflow=on
  Viterbi Decoder3 : commcnvcod2/Viterbi Decoder  trellis=poly2trellis(7, [171 133])  isPunctured=on  punctureVector=reshape([1 0;1 1],4,1)  erasures=off  dectype=Hard decision  nsdecb=4  runSigValErrCheck=off  tbdepth=34  opmode=Truncated  reset=off  delayedResetAction=off  smWordLength=16  outDataType=boolean
      settings: SourceProductName=Communications System Toolbox  SourceProductBaseCode=CM
  Out3 : Outport
  symerr : Outport  Port=2  OutputWhenDisabled=reset  InitialOutput=0
  wires:
  In3/1 -> 16-QAM Demodulator3/1, Sum/2
  16-QAM Demodulator3/1 -> Deinterleaver3/1, 16-QAM Modulator3/1
  Deinterleaver3/1 -> Viterbi Decoder3/1
  Viterbi Decoder3/1 -> RS Decoder3/1
  RS Decoder3/1 -> Out3/1
  16-QAM Modulator3/1 -> Sum/1
  Sum/1 -> symerr/1

== system ofdmexample1/Demodulator + FEC Bank/RateID4 16 QAM 3//4 ==
  In4 : Inport
  Enable : EnablePort  StatesWhenEnabling=reset  PropagateVarSize=During execution
  16-QAM Demodulator4 : commwman80216d_lib/16-QAM Demodulator  SystemSampleTime=-1
      settings: SourceProductName=Communications System Toolbox  SourceProductBaseCode=CM
  16-QAM Modulator4 : commwman80216d_lib/16-QAM Modulator  SystemSampleTime=-1
      settings: SourceProductName=Communications System Toolbox  SourceProductBaseCode=CM
  Deinterleaver4 : commwman80216d_lib/Deinterleaver  numSubCh=16  Ncbps1=768  Ncbps2=96  Ncbps3=48  Ncbps4=24  Ncbps5=12  Ncpc=4  numSym=prm80216d.numOFDMSymbols
      settings: SourceProductName=Communications System Toolbox  SourceProductBaseCode=CM
  RS Decoder4 : commwman80216d_lib/RS Decoder  N=80  K=72  numSym=prm80216d.numOFDMSymbols
      settings: SourceProductName=Communications System Toolbox  SourceProductBaseCode=CM
  Sum : Sum  Inputs=|+-  SaturateOnIntegerOverflow=on
  Viterbi Decoder4 : commcnvcod2/Viterbi Decoder  trellis=poly2trellis(7, [171 133])  isPunctured=on  punctureVector=reshape([1 0 1 0 1;1 1 0 1 0],10,1)  erasures=off  dectype=Hard decision  nsdecb=4  runSigValErrCheck=off  tbdepth=34  opmode=Truncated  reset=off  delayedResetAction=off  smWordLength=16  outDataType=boolean
      settings: SourceProductName=Communications System Toolbox  SourceProductBaseCode=CM
  Out4 : Outport
  symerr : Outport  Port=2  OutputWhenDisabled=reset  InitialOutput=0
  wires:
  In4/1 -> 16-QAM Demodulator4/1, Sum/2
  16-QAM Demodulator4/1 -> Deinterleaver4/1, 16-QAM Modulator4/1
  Deinterleaver4/1 -> Viterbi Decoder4/1
  Viterbi Decoder4/1 -> RS Decoder4/1
  RS Decoder4/1 -> Out4/1
  Sum/1 -> symerr/1
  16-QAM Modulator4/1 -> Sum/1

== system ofdmexample1/Demodulator + FEC Bank/RateID5 64QAM 2//3 ==
  In5 : Inport
  Enable : EnablePort  StatesWhenEnabling=reset  PropagateVarSize=During execution
  64-QAM Demodulator5 : commwman80216d_lib/64-QAM Demodulator  SystemSampleTime=-1
      settings: SourceProductName=Communications System Toolbox  SourceProductBaseCode=CM
  64-QAM Modulator5 : commwman80216d_lib/64-QAM Modulator  SystemSampleTime=-1
      settings: SourceProductName=Communications System Toolbox  SourceProductBaseCode=CM
  Deinterleaver5 : commwman80216d_lib/Deinterleaver  numSubCh=16  Ncbps1=1152  Ncbps2=96  Ncbps3=48  Ncbps4=24  Ncbps5=12  Ncpc=6  numSym=prm80216d.numOFDMSymbols
      settings: SourceProductName=Communications System Toolbox  SourceProductBaseCode=CM
  RS Decoder5 : commwman80216d_lib/RS Decoder  N=108  K=96  numSym=prm80216d.numOFDMSymbols
      settings: SourceProductName=Communications System Toolbox  SourceProductBaseCode=CM
  Sum : Sum  Inputs=|+-  SaturateOnIntegerOverflow=on
  Viterbi Decoder5 : commcnvcod2/Viterbi Decoder  trellis=poly2trellis(7, [171 133])  isPunctured=on  punctureVector=reshape([1 0 1;1 1 0 ],6,1)  erasures=off  dectype=Hard decision  nsdecb=4  runSigValErrCheck=off  tbdepth=34  opmode=Truncated  reset=off  delayedResetAction=off  smWordLength=16  outDataType=boolean
      settings: SourceProductName=Communications System Toolbox  SourceProductBaseCode=CM
  Out5 : Outport
  symerr : Outport  Port=2  OutputWhenDisabled=reset  InitialOutput=0
  wires:
  In5/1 -> 64-QAM Demodulator5/1, Sum/2
  64-QAM Demodulator5/1 -> Deinterleaver5/1, 64-QAM Modulator5/1
  Deinterleaver5/1 -> Viterbi Decoder5/1
  Viterbi Decoder5/1 -> RS Decoder5/1
  RS Decoder5/1 -> Out5/1
  Sum/1 -> symerr/1
  64-QAM Modulator5/1 -> Sum/1

== system ofdmexample1/Demodulator + FEC Bank/RateID6 64QAM 3//4 ==
  In6 : Inport
  Enable : EnablePort  StatesWhenEnabling=reset  PropagateVarSize=During execution
  64-QAM Demodulator6 : commwman80216d_lib/64-QAM Demodulator  SystemSampleTime=-1
      settings: SourceProductName=Communications System Toolbox  SourceProductBaseCode=CM
  64-QAM Modulator6 : commwman80216d_lib/64-QAM Modulator  SystemSampleTime=-1
      settings: SourceProductName=Communications System Toolbox  SourceProductBaseCode=CM
  Deinterleaver6 : commwman80216d_lib/Deinterleaver  numSubCh=16  Ncbps1=1152  Ncbps2=96  Ncbps3=48  Ncbps4=24  Ncbps5=12  Ncpc=6  numSym=prm80216d.numOFDMSymbols
      settings: SourceProductName=Communications System Toolbox  SourceProductBaseCode=CM
  RS Decoder6 : commwman80216d_lib/RS Decoder  N=120  K=108  numSym=prm80216d.numOFDMSymbols
      settings: SourceProductName=Communications System Toolbox  SourceProductBaseCode=CM
  Sum : Sum  Inputs=|+-  SaturateOnIntegerOverflow=on
  Viterbi Decoder6 : commcnvcod2/Viterbi Decoder  trellis=poly2trellis(7, [171 133])  isPunctured=on  punctureVector=reshape([1 0 1 0 1;1 1 0 1 0], 10, 1)  erasures=off  dectype=Hard decision  nsdecb=4  runSigValErrCheck=off  tbdepth=34  opmode=Truncated  reset=off  delayedResetAction=off  smWordLength=16  outDataType=boolean
      settings: SourceProductName=Communications System Toolbox  SourceProductBaseCode=CM
  Out6 : Outport
  symerr : Outport  Port=2  OutputWhenDisabled=reset  InitialOutput=0
  wires:
  In6/1 -> 64-QAM Demodulator6/1, Sum/2
  64-QAM Demodulator6/1 -> Deinterleaver6/1, 64-QAM Modulator6/1
  Deinterleaver6/1 -> Viterbi Decoder6/1
  Viterbi Decoder6/1 -> RS Decoder6/1
  RS Decoder6/1 -> Out6/1
  Sum/1 -> symerr/1
  64-QAM Modulator6/1 -> Sum/1

== system ofdmexample1/Digital Pre-distortion and Amplifier/Digital Pre-Distortion ==
  In1 : Inport
  In2 : Inport  Port=2
  Distortion compensation : Subsystem
  Parameter Estimation : Subsystem
  Out1 : Outport
  wires:
  In1/1 -> Distortion compensation/3(In), Parameter Estimation/1(DUT Input)
  Parameter Estimation/1(c) -> Distortion compensation/1(c)
  Parameter Estimation/2(d) -> Distortion compensation/2(d)
  Distortion compensation/1(Pre-distorted Signal) -> Out1/1
  In2/1 -> Parameter Estimation/2(DUT Output)

== system ofdmexample1/Digital Pre-distortion and Amplifier/Input//Output of Amplifier Ant ==
  DUT in : Inport
  DUT out : Inport  Port=2
  AM/AM Plot : ConstellationDiagram  Tag=ScatterPlot
  AM/PM Plot : ConstellationDiagram  Tag=ScatterPlot
  Add : Sum  Inputs=-+
  Complex to Magnitude-Angle : ComplexToMagnitudeAngle
  Complex to Magnitude-Angle1 : ComplexToMagnitudeAngle
  Real-Imag to Complex : RealImagToComplex
  Real-Imag to Complex1 : RealImagToComplex
  Unwrap : dspsigops/Unwrap  tol=pi  InputProcessing=Columns as channels (frame based)  running=on
  wires:
  Complex to Magnitude-Angle/1 -> Real-Imag to Complex/1, Real-Imag to Complex1/1
  Complex to Magnitude-Angle1/1 -> Real-Imag to Complex/2
  Real-Imag to Complex/1 -> AM/AM Plot/1
  Real-Imag to Complex1/1 -> AM/PM Plot/1
  DUT in/1 -> Complex to Magnitude-Angle/1
  DUT out/1 -> Complex to Magnitude-Angle1/1
  Complex to Magnitude-Angle1/2 -> Add/2
  Complex to Magnitude-Angle/2 -> Add/1
  Add/1 -> Unwrap/1
  Unwrap/1 -> Real-Imag to Complex1/2

== system ofdmexample1/Digital Pre-distortion and Amplifier/No nonlinearity or DPD ==
  In1 : Inport
  Action Port : ActionPort  ActionType=case
  Out1 : Outport
  wires:
  In1/1 -> Out1/1

== system ofdmexample1/Digital Pre-distortion and Amplifier/Nonlinearity with DPD ==
  In1 : Inport
  Action Port : ActionPort  ActionType=case
  Out1 : Outport
  wires:
  In1/1 -> Out1/1

== system ofdmexample1/Digital Pre-distortion and Amplifier/Only nonlinearity ==
  In1 : Inport
  Action Port : ActionPort  ActionType=case
  Out1 : Outport
  wires:
  In1/1 -> Out1/1

== system ofdmexample1/FEC & Modulator Bank/RateID0 - BPSK 1//2 ==
  In1 : Inport
  Enable : EnablePort  PropagateVarSize=During execution
  BPSK Modulator : commdigbbndpm3/BPSK Modulator Baseband  Ph=0  outDtype=double  outWordLen=16  outUDDataType=sfix(16)  outFracLenMode=Best precision  outFracLen=15  outDataTypeStr=double  outLastDataTypeStr=double
  Convolutional Encoder : commcnvcod2/Convolutional Encoder  trellis=poly2trellis(7, [171 133])  opMode=Truncated (reset every frame)  DelayedResetAction=off  hasIniStPort=off  hasFinStPort=off  usePuncVector=off  punctureVector=[1 0 1]  reset=Unused parameter value
      settings: SourceProductName=Communications System Toolbox  SourceProductBaseCode=CM
  Interleaver : commwman80216d_lib/Interleaver  numSubCh=16  Ncbps1=192  Ncbps2=96  Ncbps3=48  Ncbps4=96  Ncbps5=12  Ncpc=1  numSym=prm80216d.numOFDMSymbols
      settings: SourceProductName=Communications System Toolbox  SourceProductBaseCode=CM
  Select Bits : dspsigops/Pad  padAlong=Columns  dimsToPad=1  valSrc=Specify via dialog  padVal=0  spec=Output size  padNumOutRowsSpecMethod=User-specified  numOutRows=prm80216d.uncBlkSize(1)*8*prm80216d.numOFDMSymbols - 8  padNumOutColsSpecMethod=User-specified  numOutCols=1  isVarDimsMode=off  padBeginning=0  padEnd=0  outSizeMode=User-specified  outSize=1  padSigAt=End  trunc_flag=None  roundingMode=Floor  overflowMode=off  truncOrWrapMode=Truncate  wrap_flag=None
      settings: AttributesFormatString=\n  SourceProductName=DSP System Toolbox  SourceProductBaseCode=DS
  Zero pad tail byte : dspsigops/Pad  padAlong=Columns  dimsToPad=1  valSrc=Specify via dialog  padVal=0  spec=Output size  padNumOutRowsSpecMethod=User-specified  numOutRows=prm80216d.uncBlkSize(1)*8*prm80216d.numOFDMSymbols  padNumOutColsSpecMethod=User-specified  numOutCols=1  isVarDimsMode=off  padBeginning=0  padEnd=0  outSizeMode=User-specified  outSize=1  padSigAt=End  trunc_flag=None  roundingMode=Floor  overflowMode=off  truncOrWrapMode=Truncate  wrap_flag=None
      settings: AttributesFormatString=\n  SourceProductName=DSP System Toolbox  SourceProductBaseCode=DS
  Out1 : Outport
  wires:
  Convolutional Encoder/1 -> Interleaver/1
  Interleaver/1 -> BPSK Modulator/1
  In1/1 -> Select Bits/1
  BPSK Modulator/1 -> Out1/1
  Select Bits/1 -> Zero pad tail byte/1
  Zero pad tail byte/1 -> Convolutional Encoder/1

== system ofdmexample1/FEC & Modulator Bank/RateID1 - QPSK 1//2 ==
  In1 : Inport
  Enable : EnablePort  PropagateVarSize=During execution
  Interleaver1 : commwman80216d_lib/Interleaver  numSubCh=16  Ncbps1=384  Ncbps2=96  Ncbps3=48  Ncbps4=96  Ncbps5=12  Ncpc=2  numSym=prm80216d.numOFDMSymbols
      settings: SourceProductName=Communications System Toolbox  SourceProductBaseCode=CM
  Punctured Convolutional Encoder1 : commcnvcod2/Convolutional Encoder  trellis=poly2trellis(7, [171 133])  opMode=Truncated (reset every frame)  DelayedResetAction=off  hasIniStPort=off  hasFinStPort=off  usePuncVector=on  punctureVector=reshape([1 0;1 1],4,1)  reset=Unused parameter value
      settings: SourceProductName=Communications System Toolbox  SourceProductBaseCode=CM
  QPSK Modulator1 : commwman80216d_lib/QPSK Modulator  SystemSampleTime=-1
      settings: SourceProductName=Communications System Toolbox  SourceProductBaseCode=CM
  RS Encoder1 : commwman80216d_lib/RS Encoder  N=32  K=24  numSym=prm80216d.numOFDMSymbols
      settings: SourceProductName=Communications System Toolbox  SourceProductBaseCode=CM
  Select Bits : dspsigops/Pad  padAlong=Columns  dimsToPad=1  valSrc=Specify via dialog  padVal=0  spec=Output size  padNumOutRowsSpecMethod=User-specified  numOutRows=prm80216d.uncBlkSize(2)*8*prm80216d.numOFDMSymbols - 8  padNumOutColsSpecMethod=User-specified  numOutCols=1  isVarDimsMode=off  padBeginning=0  padEnd=0  outSizeMode=User-specified  outSize=1  padSigAt=End  trunc_flag=None  roundingMode=Floor  overflowMode=off  truncOrWrapMode=Truncate  wrap_flag=None
      settings: AttributesFormatString=\n  SourceProductName=DSP System Toolbox  SourceProductBaseCode=DS
  Zero pad tail byte : dspsigops/Pad  padAlong=Columns  dimsToPad=1  valSrc=Specify via dialog  padVal=0  spec=Output size  padNumOutRowsSpecMethod=User-specified  numOutRows=prm80216d.uncBlkSize(2)*8*prm80216d.numOFDMSymbols  padNumOutColsSpecMethod=User-specified  numOutCols=1  isVarDimsMode=off  padBeginning=0  padEnd=0  outSizeMode=User-specified  outSize=1  padSigAt=End  trunc_flag=None  roundingMode=Floor  overflowMode=off  truncOrWrapMode=Truncate  wrap_flag=None
      settings: AttributesFormatString=\n  SourceProductName=DSP System Toolbox  SourceProductBaseCode=DS
  Out1 : Outport
  wires:
  RS Encoder1/1 -> Punctured Convolutional Encoder1/1
  Punctured Convolutional Encoder1/1 -> Interleaver1/1
  Interleaver1/1 -> QPSK Modulator1/1
  In1/1 -> Select Bits/1
  QPSK Modulator1/1 -> Out1/1
  Select Bits/1 -> Zero pad tail byte/1
  Zero pad tail byte/1 -> RS Encoder1/1

== system ofdmexample1/FEC & Modulator Bank/RateID2 - QPSK 3//4 ==
  In1 : Inport
  Enable : EnablePort  PropagateVarSize=During execution
  Interleaver2 : commwman80216d_lib/Interleaver  numSubCh=16  Ncbps1=384  Ncbps2=96  Ncbps3=48  Ncbps4=96  Ncbps5=12  Ncpc=2  numSym=prm80216d.numOFDMSymbols
      settings: SourceProductName=Communications System Toolbox  SourceProductBaseCode=CM
  Punctured Convolutional Encoder2 : commcnvcod2/Convolutional Encoder  trellis=poly2trellis(7, [171 133])  opMode=Truncated (reset every frame)  DelayedResetAction=off  hasIniStPort=off  hasFinStPort=off  usePuncVector=on  punctureVector=reshape([1 0 1 0 1;1 1 0 1 0],10,1)  reset=Unused parameter value
      settings: SourceProductName=Communications System Toolbox  SourceProductBaseCode=CM
  QPSK Modulator2 : commwman80216d_lib/QPSK Modulator  SystemSampleTime=-1
      settings: SourceProductName=Communications System Toolbox  SourceProductBaseCode=CM
  RS Encoder2 : commwman80216d_lib/RS Encoder  N=40  K=36  numSym=prm80216d.numOFDMSymbols
      settings: SourceProductName=Communications System Toolbox  SourceProductBaseCode=CM
  Select Bits : dspsigops/Pad  padAlong=Columns  dimsToPad=1  valSrc=Specify via dialog  padVal=0  spec=Output size  padNumOutRowsSpecMethod=User-specified  numOutRows=prm80216d.uncBlkSize(3)*8*prm80216d.numOFDMSymbols - 8  padNumOutColsSpecMethod=User-specified  numOutCols=1  isVarDimsMode=off  padBeginning=0  padEnd=0  outSizeMode=User-specified  outSize=1  padSigAt=End  trunc_flag=None  roundingMode=Floor  overflowMode=off  truncOrWrapMode=Truncate  wrap_flag=None
      settings: AttributesFormatString=\n  SourceProductName=DSP System Toolbox  SourceProductBaseCode=DS
  Zero pad tail byte : dspsigops/Pad  padAlong=Columns  dimsToPad=1  valSrc=Specify via dialog  padVal=0  spec=Output size  padNumOutRowsSpecMethod=User-specified  numOutRows=prm80216d.uncBlkSize(3)*8*prm80216d.numOFDMSymbols  padNumOutColsSpecMethod=User-specified  numOutCols=1  isVarDimsMode=off  padBeginning=0  padEnd=0  outSizeMode=User-specified  outSize=1  padSigAt=End  trunc_flag=None  roundingMode=Floor  overflowMode=off  truncOrWrapMode=Truncate  wrap_flag=None
      settings: AttributesFormatString=\n  SourceProductName=DSP System Toolbox  SourceProductBaseCode=DS
  Out1 : Outport
  wires:
  RS Encoder2/1 -> Punctured Convolutional Encoder2/1
  Punctured Convolutional Encoder2/1 -> Interleaver2/1
  Interleaver2/1 -> QPSK Modulator2/1
  In1/1 -> Select Bits/1
  QPSK Modulator2/1 -> Out1/1
  Select Bits/1 -> Zero pad tail byte/1
  Zero pad tail byte/1 -> RS Encoder2/1

== system ofdmexample1/FEC & Modulator Bank/RateID3 - 16QAM 1//2 ==
  In1 : Inport
  Enable : EnablePort  PropagateVarSize=During execution
  16-QAM Modulator3 : commwman80216d_lib/16-QAM Modulator  SystemSampleTime=-1
      settings: SourceProductName=Communications System Toolbox  SourceProductBaseCode=CM
  Interleaver3 : commwman80216d_lib/Interleaver  numSubCh=16  Ncbps1=768  Ncbps2=96  Ncbps3=48  Ncbps4=96  Ncbps5=12  Ncpc=4  numSym=prm80216d.numOFDMSymbols
      settings: SourceProductName=Communications System Toolbox  SourceProductBaseCode=CM
  Punctured Convolutional Encoder3 : commcnvcod2/Convolutional Encoder  trellis=poly2trellis(7, [171 133])  opMode=Truncated (reset every frame)  DelayedResetAction=off  hasIniStPort=off  hasFinStPort=off  usePuncVector=on  punctureVector=reshape([1 0;1 1],4,1)  reset=Unused parameter value
      settings: SourceProductName=Communications System Toolbox  SourceProductBaseCode=CM
  RS Encoder3 : commwman80216d_lib/RS Encoder  N=64  K=48  numSym=prm80216d.numOFDMSymbols
      settings: SourceProductName=Communications System Toolbox  SourceProductBaseCode=CM
  Select Bits : dspsigops/Pad  padAlong=Columns  dimsToPad=1  valSrc=Specify via dialog  padVal=0  spec=Output size  padNumOutRowsSpecMethod=User-specified  numOutRows=prm80216d.uncBlkSize(4)*8*prm80216d.numOFDMSymbols - 8  padNumOutColsSpecMethod=User-specified  numOutCols=1  isVarDimsMode=off  padBeginning=0  padEnd=0  outSizeMode=User-specified  outSize=1  padSigAt=End  trunc_flag=None  roundingMode=Floor  overflowMode=off  truncOrWrapMode=Truncate  wrap_flag=None
      settings: AttributesFormatString=\n  SourceProductName=DSP System Toolbox  SourceProductBaseCode=DS
  Zero pad tail byte : dspsigops/Pad  padAlong=Columns  dimsToPad=1  valSrc=Specify via dialog  padVal=0  spec=Output size  padNumOutRowsSpecMethod=User-specified  numOutRows=prm80216d.uncBlkSize(4)*8*prm80216d.numOFDMSymbols  padNumOutColsSpecMethod=User-specified  numOutCols=1  isVarDimsMode=off  padBeginning=0  padEnd=0  outSizeMode=User-specified  outSize=1  padSigAt=End  trunc_flag=None  roundingMode=Floor  overflowMode=off  truncOrWrapMode=Truncate  wrap_flag=None
      settings: AttributesFormatString=\n  SourceProductName=DSP System Toolbox  SourceProductBaseCode=DS
  Out1 : Outport
  wires:
  RS Encoder3/1 -> Punctured Convolutional Encoder3/1
  Punctured Convolutional Encoder3/1 -> Interleaver3/1
  Interleaver3/1 -> 16-QAM Modulator3/1
  In1/1 -> Select Bits/1
  16-QAM Modulator3/1 -> Out1/1
  Select Bits/1 -> Zero pad tail byte/1
  Zero pad tail byte/1 -> RS Encoder3/1

== system ofdmexample1/FEC & Modulator Bank/RateID4 - 16QAM 3//4 ==
  In1 : Inport
  Enable : EnablePort  PropagateVarSize=During execution
  16-QAM Modulator4 : commwman80216d_lib/16-QAM Modulator  SystemSampleTime=-1
      settings: SourceProductName=Communications System Toolbox  SourceProductBaseCode=CM
  Interleaver4 : commwman80216d_lib/Interleaver  numSubCh=16  Ncbps1=768  Ncbps2=96  Ncbps3=48  Ncbps4=96  Ncbps5=12  Ncpc=4  numSym=prm80216d.numOFDMSymbols
      settings: SourceProductName=Communications System Toolbox  SourceProductBaseCode=CM
  Punctured Convolutional Encoder4 : commcnvcod2/Convolutional Encoder  trellis=poly2trellis(7, [171 133])  opMode=Truncated (reset every frame)  DelayedResetAction=off  hasIniStPort=off  hasFinStPort=off  usePuncVector=on  punctureVector=reshape([1 0 1 0 1;1 1 0 1 0],10,1)  reset=Unused parameter value
      settings: SourceProductName=Communications System Toolbox  SourceProductBaseCode=CM
  RS Encoder4 : commwman80216d_lib/RS Encoder  N=80  K=72  numSym=prm80216d.numOFDMSymbols
      settings: SourceProductName=Communications System Toolbox  SourceProductBaseCode=CM
  Select Bits : dspsigops/Pad  padAlong=Columns  dimsToPad=1  valSrc=Specify via dialog  padVal=0  spec=Output size  padNumOutRowsSpecMethod=User-specified  numOutRows=prm80216d.uncBlkSize(5)*8*prm80216d.numOFDMSymbols - 8  padNumOutColsSpecMethod=User-specified  numOutCols=1  isVarDimsMode=off  padBeginning=0  padEnd=0  outSizeMode=User-specified  outSize=1  padSigAt=End  trunc_flag=None  roundingMode=Floor  overflowMode=off  truncOrWrapMode=Truncate  wrap_flag=None
      settings: AttributesFormatString=\n  SourceProductName=DSP System Toolbox  SourceProductBaseCode=DS
  Zero pad tail byte : dspsigops/Pad  padAlong=Columns  dimsToPad=1  valSrc=Specify via dialog  padVal=0  spec=Output size  padNumOutRowsSpecMethod=User-specified  numOutRows=prm80216d.uncBlkSize(5)*8*prm80216d.numOFDMSymbols  padNumOutColsSpecMethod=User-specified  numOutCols=1  isVarDimsMode=off  padBeginning=0  padEnd=0  outSizeMode=User-specified  outSize=1  padSigAt=End  trunc_flag=None  roundingMode=Floor  overflowMode=off  truncOrWrapMode=Truncate  wrap_flag=None
      settings: AttributesFormatString=\n  SourceProductName=DSP System Toolbox  SourceProductBaseCode=DS
  Out1 : Outport
  wires:
  RS Encoder4/1 -> Punctured Convolutional Encoder4/1
  Punctured Convolutional Encoder4/1 -> Interleaver4/1
  Interleaver4/1 -> 16-QAM Modulator4/1
  In1/1 -> Select Bits/1
  16-QAM Modulator4/1 -> Out1/1
  Select Bits/1 -> Zero pad tail byte/1
  Zero pad tail byte/1 -> RS Encoder4/1
